simulink model "conroltanquesconvariadorvelocidad2"  (Simulink 5.0)
settings: Solver=ode5  StartTime=0.0  StopTime=inf  FixedStep=0.125  RelTol=1e-3
libraries: simulink x2
settings Model: LastModifiedBy=XPMUser  RTWOptions="-aEnforceIntegerDowncast=1 -aExtMode=0 -aExtModeTesting=0 -aFoldNonRolledExpr=1 -aForceParamTrailComments=0 -aGenerateComments=1 -aGenerateReport=0 -aIgnoreCustomStorageClasses=1 -aIncDataTypeInIds=0 -aIncHierarchyInIds=0 -aInlineInvariantSignals=1 -aInlineParameters=0 -aInlinedPrmAccess=\"Literals\" -aLocalBlockOutputs=1 -aLogVarNameModifier=\"rt_\" -aMaxRTWIdLen=31 -aPrefixModelToSubsysFcnNames=1 -aRTWVerbose=1 -aRollThreshold=5 -aShowEliminatedStatements=0"

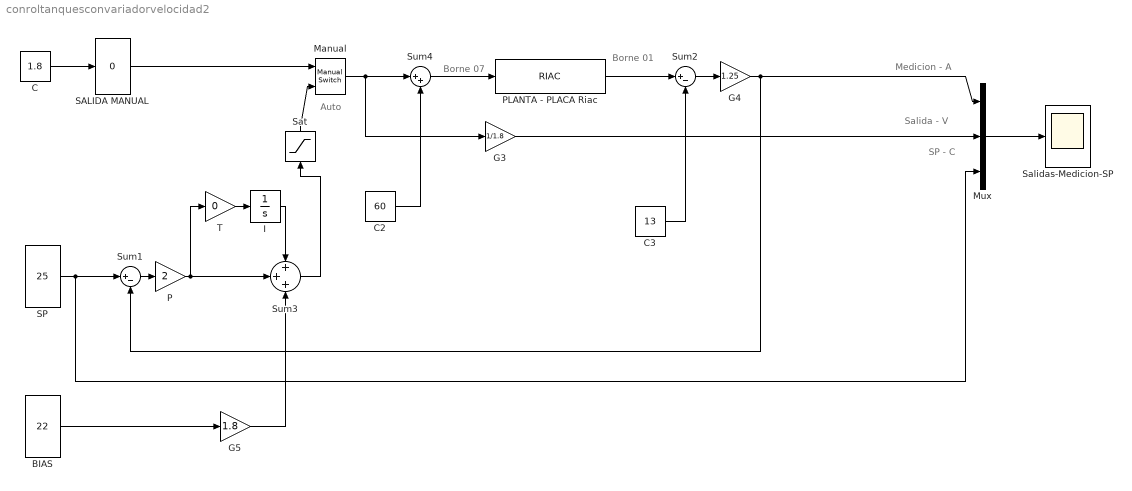
== system conroltanquesconvariadorvelocidad2 ==
  note: Auto
  note: Medicion - A
  note: Salida - V
  note: SP - C
  note: Borne 07
  note: Borne 01
  " SALIDA MANUAL" : simulink/Math Operations/Slider Gain  low=0  gain=0  high=100
  BIAS : Constant  Value=22  VectorParams1D=off
  C : Constant  Value=1.8  VectorParams1D=off
  C2 : Constant  Value=60  VectorParams1D=off
  C3 : Constant  Value=13  VectorParams1D=off
  G3 : Gain  Gain=1/1.8  SaturateOnIntegerOverflow=on
  G4 : Gain  Gain=1.25  SaturateOnIntegerOverflow=on
  G5 : Gain  Gain=1.8  SaturateOnIntegerOverflow=on
  I : Integrator  LimitOutput=on  UpperSaturationLimit=180  LowerSaturationLimit=-180
  "Manual " : simulink/Signal Routing/Manual Switch  sw=1  action=0
  Mux : Mux  Inputs=3
  P : Gain  Gain=2  SaturateOnIntegerOverflow=on
  PLANTA - PLACA Riac : S-Function  FunctionName=RIAC
  SP : Constant  Value=25  VectorParams1D=off
  Salidas-Medicion-SP : Scope
      settings: TimeRange=300  YMin=0  YMax=100
  Sat : Saturate  Orientation=up  UpperLimit=180  LowerLimit=0
  Sum1 : Sum  Inputs=|+-  SaturateOnIntegerOverflow=on
  Sum2 : Sum  Inputs=|+-  SaturateOnIntegerOverflow=on
  Sum3 : Sum  Inputs=+++  SaturateOnIntegerOverflow=on
  Sum4 : Sum  Inputs=|++  SaturateOnIntegerOverflow=on
  T : Gain  Gain=0  SaturateOnIntegerOverflow=on
  wires:
  Mux/1 -> Salidas-Medicion-SP/1
  " SALIDA MANUAL"/1 -> "Manual "/1
  SP/1 -> Sum1/1, Mux/3
  BIAS/1 -> G5/1
  Sat/1 -> "Manual "/2
  PLANTA - PLACA Riac/1 -> Sum2/1
  Sum2/1 -> G4/1
  G4/1 -> Mux/1, Sum1/2
  C3/1 -> Sum2/2
  "Manual "/1 -> Sum4/1, G3/1
  C2/1 -> Sum4/2
  Sum4/1 -> PLANTA - PLACA Riac/1
  G3/1 -> Mux/2
  C/1 -> " SALIDA MANUAL"/1
  Sum1/1 -> P/1
  Sum3/1 -> Sat/1
  G5/1 -> Sum3/3
  I/1 -> Sum3/1
  T/1 -> I/1
  P/1 -> Sum3/2, T/1
